simulink model "Three_Phase_inverter"  (R2019a)
settings: Solver=VariableStepAuto  StartTime=0.0  StopTime=0.009  RelTol=1e-3
libraries: powerlib x15
settings Model: Creator=Utkarsh  LastModifiedBy=Utkarsh

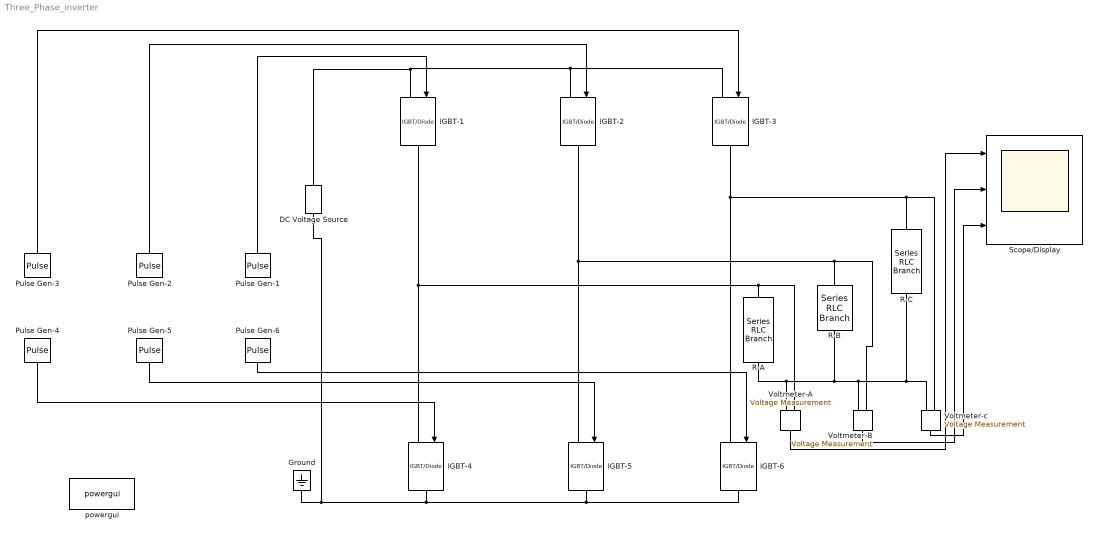
== system Three_Phase_inverter ==
  DC Voltage Source : powerlib/Electrical Sources/DC Voltage Source  Amplitude=100  Measurements=None
      settings: SourceProductName=Simscape Electrical
  Ground : powerlib/Elements/Ground  LConnTagsString=a
      settings: SourceProductName=Simscape Electrical
  IGBT-{1..6} (6 alike) : powerlib/Power Electronics/IGBT//Diode  Ron=1e-3  Rs=1e5  Cs=inf  Measurements=off
      settings: SourceProductName=Simscape Electrical
  Pulse Gen-1 : DiscretePulseGenerator  PulseType=Time based  Amplitude=20  Period=6e-4  PulseWidth=50
  Pulse Gen-2 : DiscretePulseGenerator  PulseType=Time based  Amplitude=20  Period=6e-4  PulseWidth=50  PhaseDelay=2e-4
  Pulse Gen-3 : DiscretePulseGenerator  PulseType=Time based  Amplitude=20  Period=6e-4  PulseWidth=50  PhaseDelay=4e-4
  Pulse Gen-4 : DiscretePulseGenerator  PulseType=Time based  Amplitude=20  Period=6e-4  PulseWidth=50  PhaseDelay=3e-4
  Pulse Gen-5 : DiscretePulseGenerator  PulseType=Time based  Amplitude=20  Period=6e-4  PulseWidth=50  PhaseDelay=5e-4
  Pulse Gen-6 : DiscretePulseGenerator  PulseType=Time based  Amplitude=20  Period=6e-4  PulseWidth=50  PhaseDelay=1e-4
  R-A : powerlib/Elements/Series RLC Branch  LConnTagsString=__new0  RConnTagsString=__new0  BranchType=R  Resistance=1000  Inductance=1e-3  SetiL0=off  InitialCurrent=0  Capacitance=1e-6  Setx0=off  InitialVoltage=0  Measurements=None
      settings: SourceProductName=Simscape Electrical
  R-B : powerlib/Elements/Series RLC Branch  LConnTagsString=__new0  RConnTagsString=__new0  BranchType=R  Resistance=1000  Inductance=1e-3  SetiL0=off  InitialCurrent=0  Capacitance=1e-6  Setx0=off  InitialVoltage=0  Measurements=None
      settings: SourceProductName=Simscape Electrical
  R-C : powerlib/Elements/Series RLC Branch  LConnTagsString=__new0  RConnTagsString=__new0  BranchType=R  Resistance=1000  Inductance=1e-3  SetiL0=off  InitialCurrent=0  Capacitance=1e-6  Setx0=off  InitialVoltage=0  Measurements=None
      settings: SourceProductName=Simscape Electrical
  Scope/Display : Scope  NumInputPorts=3
  Voltmeter-A : powerlib/Measurements/Voltage Measurement  PhasorSimulation=off  OutputType=Complex  PSBequivalent=0
      settings: SourceProductName=Simscape Electrical
  Voltmeter-B : powerlib/Measurements/Voltage Measurement  PhasorSimulation=off  OutputType=Complex  PSBequivalent=0
      settings: SourceProductName=Simscape Electrical
  Voltmeter-c : powerlib/Measurements/Voltage Measurement  PhasorSimulation=off  OutputType=Complex  PSBequivalent=0
      settings: SourceProductName=Simscape Electrical
  powergui : powerlib/powergui  Priority=1  SimulationMode=Continuous  SampleTime=50e-6  frequency=60  Iterations=50  frequencyindice=0  Pbase=100e6  ErrMax=1e-4  UnitsV=kV  UnitsW=MW  buscounter=0  FunctionMessages=off  echomessages=off  EnableUseOfTLC=off  CurrentSourceSwitches=off  DisableSnubberDevices=off  DisableRonSwitches=off  DisableVfSwitches=off  DisplayEquations=off  AutomaticDiscreteSolvers=off  SolverType=Tustin/Backward Euler (TBE)  Interpol=off  ExternalGateDelay=off  methode=off  Ts=100  x0status=blocks  SPID=on  SwTol=0  HookPort=off  NonlinearTolerance=0  nMaxIteration=15  ContinueOnMaxIteration=off  RestoreLinks=warning  ResistiveCurrentMeasurement=off  Frange=[0:2:500]  Ylog=off  Xlog=on  ShowGrid=off  save=off  variable=ZData  structure=0  ZoomFFT=off  StartTime=0.0  cycles=1  DisplayStyle=1  fundamental=60  FreqAxis=off  MaxFrequency=1000  frequencyindicesteady=1  RmsSteady=1  display=off
      settings: SourceProductName=Simscape Electrical
  wires:
  Pulse Gen-1/1 -> IGBT-1/1
  Pulse Gen-2/1 -> IGBT-2/1
  Pulse Gen-3/1 -> IGBT-3/1
  Pulse Gen-4/1 -> IGBT-4/1
  Pulse Gen-5/1 -> IGBT-5/1
  Pulse Gen-6/1 -> IGBT-6/1
  Voltmeter-A/1 -> Scope/Display/1
  Voltmeter-B/1 -> Scope/Display/2
  Voltmeter-c/1 -> Scope/Display/3
  connections:
  IGBT-5/RConn1 -- IGBT-6/RConn1 -- Ground/LConn1 -- DC Voltage Source/LConn1 -- IGBT-4/RConn1
  IGBT-3/LConn1 -- IGBT-2/LConn1 -- DC Voltage Source/RConn1 -- IGBT-1/LConn1
  IGBT-2/RConn1 -- IGBT-5/LConn1 -- Voltmeter-B/LConn1 -- R-B/RConn1
  IGBT-1/RConn1 -- IGBT-4/LConn1 -- Voltmeter-A/LConn1 -- R-A/LConn1
  IGBT-3/RConn1 -- Voltmeter-c/LConn1 -- R-C/RConn1 -- IGBT-6/LConn1
  R-A/RConn1 -- Voltmeter-A/LConn2 -- Voltmeter-c/LConn2 -- R-C/LConn1 -- Voltmeter-B/LConn2 -- R-B/LConn1
